simulink model "pratica11S"  (R2021b)
settings: Solver=VariableStepAuto  StartTime=0.0  StopTime=24.00  RelTol=1e-3
values from neighbouring files (symbols this model uses):
  R = 1.15    [pratica11.m]
  T0 = (2*pi)/ws    [pratica11.m]
undefined symbols (not defined in the file or in its folder): Cd, Dc, F, H
settings Model: Creator=carlo  LastModifiedBy=carlo

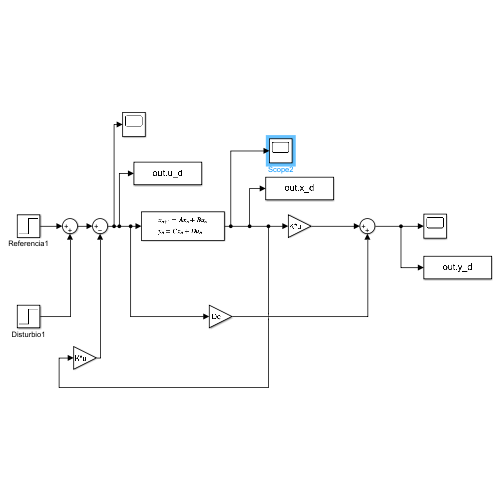
[thumbnail: Simulink's stored preview of the top-level diagram]
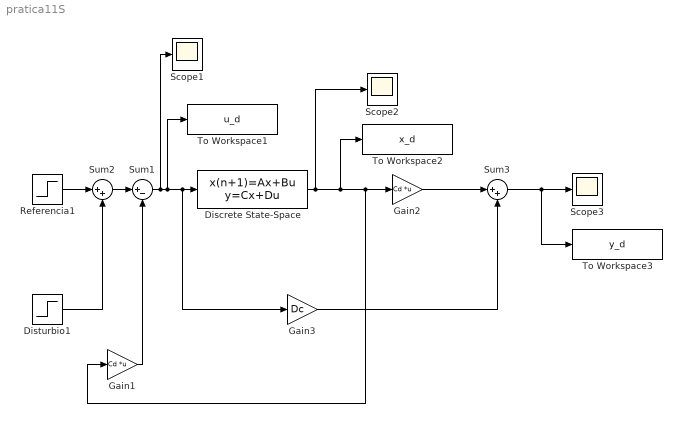
== system pratica11S ==
  Discrete State-Space : DiscreteStateSpace  A=F  B=H  C=[1 0; 0 1]  D=[0 ; 0]  SampleTime=T0
  Disturbio1 : Step  Time=0  After=R  SampleTime=0
  Gain1 : Gain  Gain=Cd  Multiplication=Matrix(K*u)
  Gain2 : Gain  Gain=Cd  Multiplication=Matrix(K*u)
  Gain3 : Gain  Gain=Dc
  Referencia1 : Step  Time=0  After=R  SampleTime=0
  Scope1 : Scope
  Scope2 : Scope
  Scope3 : Scope
  Sum1 : Sum  Inputs=|+-
  Sum2 : Sum  Inputs=|++
  Sum3 : Sum  Inputs=|++
  To Workspace1 : ToWorkspace  VariableName=u_d  SaveFormat=Timeseries  SampleTime=-1
  To Workspace2 : ToWorkspace  VariableName=x_d  SaveFormat=Timeseries  SampleTime=-1
  To Workspace3 : ToWorkspace  VariableName=y_d  SaveFormat=Timeseries  SampleTime=-1
  wires:
  Sum2/1 -> Sum1/1
  Discrete State-Space/1 -> Scope2/1, To Workspace2/1, Gain1/1, Gain2/1
  Gain3/1 -> Sum3/2
  Sum3/1 -> To Workspace3/1, Scope3/1
  Disturbio1/1 -> Sum2/2
  Referencia1/1 -> Sum2/1
  Gain2/1 -> Sum3/1
  Sum1/1 -> Scope1/1, To Workspace1/1, Gain3/1, Discrete State-Space/1
  Gain1/1 -> Sum1/2
